simulink model "UAV_3dof_Autonomus"  (R2024b)
settings: Solver=FixedStepDiscrete  StartTime=0.0  StopTime=180  FixedStep=0.05  RelTol=1e-3
settings Model: Creator=ninadbhave  LastModifiedBy=ninadbhave

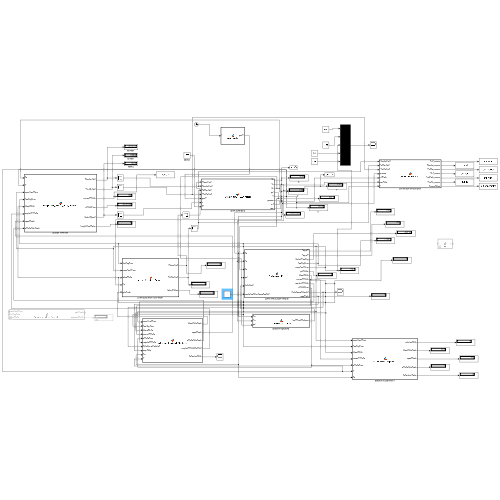
[thumbnail: Simulink's stored preview of the top-level diagram]
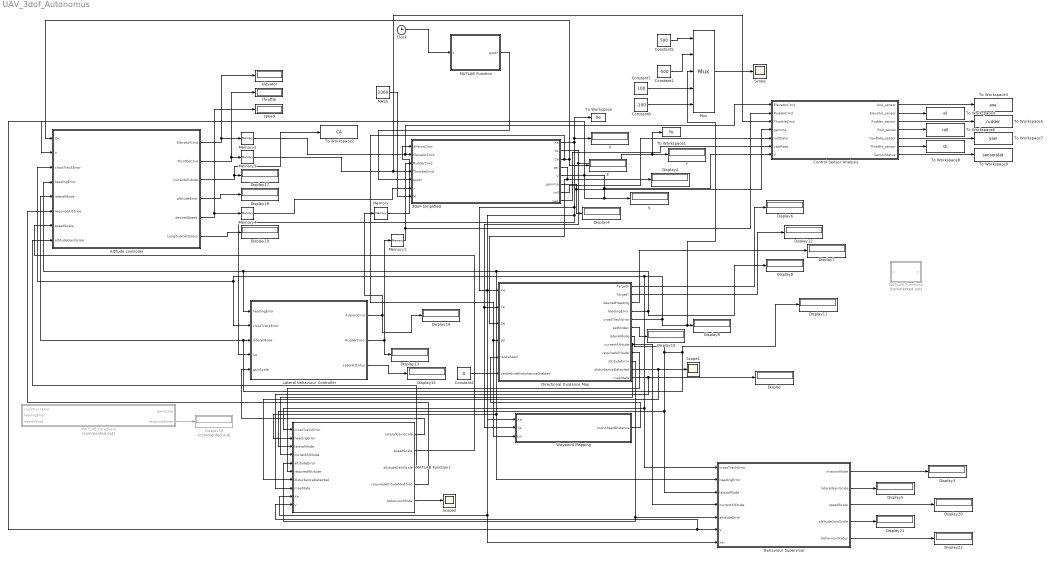
== system UAV_3dof_Autonomus ==
  3DoF-Simplified : MATLAB Function  TreatAsAtomicUnit=on
  Altitude controller : MATLAB Function  TreatAsAtomicUnit=on
  Behaviour Supervisor : MATLAB Function  TreatAsAtomicUnit=on
  Clock : Clock
  Constant1 : Constant  Value=-500
  Constant2 : Constant  Value=0
  Constant5 : Constant  Value=500
  Constant7 : Constant  Value=100
  Constant8 : Constant  Value=-100
  Control Sensor Analysis : MATLAB Function  TreatAsAtomicUnit=on
  Directional Guidance Map : MATLAB Function  TreatAsAtomicUnit=on
  Display{,2..15,17..22} (21 alike) : Display
  Display16 : Display  Commented=on
  Lateral behaviour Controller : MATLAB Function  TreatAsAtomicUnit=on
  MASS : Constant  Value=1000
  MATLAB Function : MATLAB Function  TreatAsAtomicUnit=on
  MATLAB Function1 : MATLAB Function  TreatAsAtomicUnit=on
  MATLAB Function2 : MATLAB Function  Commented=on  TreatAsAtomicUnit=on
  MATLAB Function4 : MATLAB Function  Commented=on  TreatAsAtomicUnit=on
  Memory : Memory
  Memory1 : Memory
  Memory2 : Memory  InitialCondition=-0.003
  Memory3 : Memory  InitialCondition=0.55
  Memory4 : Memory  InitialCondition=45
  Mux : Mux  Inputs=5
  Scope : Scope
  Scope1 : Scope
  Scope2 : Scope
  To Workspace : ToWorkspace  VariableName=Xe  SaveFormat=Timeseries  SampleTime=-1
  To Workspace1 : ToWorkspace  VariableName=Ye  SaveFormat=Timeseries  SampleTime=-1
  To Workspace2 : ToWorkspace  VariableName=CA  SaveFormat=Timeseries  SampleTime=-1
  To Workspace3 : ToWorkspace  VariableName=aoa  SaveFormat=Timeseries  SampleTime=-1
  To Workspace4 : ToWorkspace  VariableName=el  SaveFormat=Timeseries  SampleTime=-1
  To Workspace5 : ToWorkspace  VariableName=rudder  SaveFormat=Timeseries  SampleTime=-1
  To Workspace6 : ToWorkspace  VariableName=roll  SaveFormat=Timeseries  SampleTime=-1
  To Workspace7 : ToWorkspace  VariableName=yaw  SaveFormat=Timeseries  SampleTime=-1
  To Workspace8 : ToWorkspace  VariableName=th  SaveFormat=Timeseries  SampleTime=-1
  To Workspace9 : ToWorkspace  VariableName=sensorstat  SaveFormat=Timeseries  SampleTime=-1
  V : Display
  Waypoint Mapping : MATLAB Function  TreatAsAtomicUnit=on
  X : Display
  Y : Display
  Z : Display
  elevator : Display
  speed : Display
  throttle : Display
  wires:
  MATLAB Function/1(gustY) -> 3DoF-Simplified/5(gustY)
  3DoF-Simplified/1(Xe) -> MATLAB Function1/9(Xe), Behaviour Supervisor/7(Xe), Lateral behaviour Controller/4(Xe), Waypoint Mapping/1(Xe), Directional Guidance Map/1(Xe), To Workspace/1, X/1
  3DoF-Simplified/6(gamma) -> Display4/1, Control Sensor Analysis/4(gamma)
  3DoF-Simplified/5(V) -> MATLAB Function1/10(V), Behaviour Supervisor/6(V), Control Sensor Analysis/7(V), V/1, Altitude controller/2(V)
  3DoF-Simplified/4(psi) -> Display2/1, Waypoint Mapping/3(psi), Directional Guidance Map/4(psi)
  3DoF-Simplified/3(Ze) -> Directional Guidance Map/3(Ze), Z/1, Altitude controller/1(Ze)
  3DoF-Simplified/2(Ye) -> To Workspace1/1, Y/1, Waypoint Mapping/2(Ye), Directional Guidance Map/2(Ye)
  Directional Guidance Map/1(TargetX) -> Display6/1
  Directional Guidance Map/7(lateralMode) -> Behaviour Supervisor/3(lateralMode), MATLAB Function1/3(lateralMode), Display11/1, Altitude controller/5(lateralMode), Lateral behaviour Controller/3(lateralMode)
  Directional Guidance Map/6(pathIndex) -> Display10/1
  Directional Guidance Map/5(crossTrackError) -> Lateral behaviour Controller/2(crossTrackError), Altitude controller/3(crossTrackError), Behaviour Supervisor/1(crossTrackError), MATLAB Function1/1(crossTrackError), Mux/3, Display9/1
  Directional Guidance Map/4(headingError) -> Altitude controller/4(headingError), Lateral behaviour Controller/1(headingError), Behaviour Supervisor/2(headingError), MATLAB Function1/2(headingError), Display8/1
  Directional Guidance Map/3(desiredHeading) -> Display7/1
  Directional Guidance Map/2(TargetY) -> Display12/1
  Lateral behaviour Controller/1(AileronCmd) -> Display14/1, Memory/1
  Lateral behaviour Controller/2(RudderCmd) -> Display13/1, Memory1/1
  Memory/1 -> 3DoF-Simplified/1(AileronCmd)
  Memory1/1 -> 3DoF-Simplified/3(RudderCmd), Control Sensor Analysis/2(RudderCmd)
  Lateral behaviour Controller/3(LateralStatus) -> Display15/1
  Waypoint Mapping/1(lookAheadDistance) -> Directional Guidance Map/5(lookahead)
  Constant5/1 -> Mux/1
  Mux/1 -> Scope/1
  Constant1/1 -> Mux/2
  MATLAB Function4/2(responseMode) -> Display16/1
  Constant7/1 -> Mux/4
  Constant8/1 -> Mux/5
  Altitude controller/3(currentAltitude) -> To Workspace2/1, Display17/1
  Altitude controller/4(altitudeError) -> Display18/1
  Altitude controller/6(LongitudinalStatus) -> Display19/1
  Altitude controller/1(ElevatorCmd) -> elevator/1, Memory2/1
  Memory2/1 -> Control Sensor Analysis/1(ElevatorCmd), 3DoF-Simplified/2(ElevatorCmd)
  Altitude controller/2(ThrottleCmd) -> throttle/1, Memory3/1
  Memory3/1 -> 3DoF-Simplified/4(ThrottleCmd), Control Sensor Analysis/3(ThrottleCmd)
  Altitude controller/5(desiredSpeed) -> speed/1, Memory4/1
  Memory4/1 -> 3DoF-Simplified/6(v)
  MASS/1 -> 3DoF-Simplified/7(M)
  Clock/1 -> MATLAB Function/1(t)
  3DoF-Simplified/7(roll) -> Control Sensor Analysis/5(rollState)
  3DoF-Simplified/8(yaw) -> Control Sensor Analysis/6(yawRate)
  Control Sensor Analysis/1(AoA_sensor) -> To Workspace3/1
  Control Sensor Analysis/2(Elevator_sensor) -> To Workspace4/1
  Control Sensor Analysis/3(Rudder_sensor) -> To Workspace5/1
  Control Sensor Analysis/4(Roll_sensor) -> To Workspace6/1
  Control Sensor Analysis/5(YawRate_sensor) -> To Workspace7/1
  Control Sensor Analysis/6(Throttle_sensor) -> To Workspace8/1
  Control Sensor Analysis/7(SensorStatus) -> To Workspace9/1
  Constant2/1 -> Directional Guidance Map/6(centrelineDisturbanceEnabled)
  Directional Guidance Map/12(mapState) -> MATLAB Function1/8(mapState), Display/1
  Directional Guidance Map/8(currentAltitude) -> MATLAB Function1/4(currentAltitude), Behaviour Supervisor/4(currentAltitude)
  Directional Guidance Map/10(altitudeError) -> MATLAB Function1/5(altitudeError), Behaviour Supervisor/5(altitudeError)
  Directional Guidance Map/9(requiredAltitude) -> MATLAB Function1/6(requiredAltitude)
  Directional Guidance Map/11(disturbanceDetected) -> MATLAB Function1/7(disturbanceDetected), Scope1/1
  Behaviour Supervisor/1(missionMode) -> Display3/1
  Behaviour Supervisor/2(lateralGainScale) -> Display5/1
  Behaviour Supervisor/3(speedScale) -> Display20/1
  Behaviour Supervisor/4(altitudeGainScale) -> Display21/1
  Behaviour Supervisor/5(behaviourStatus) -> Display22/1
  MATLAB Function1/1(lateralGainScale) -> Lateral behaviour Controller/5(gainScale)
  MATLAB Function1/4(requiredAltitudeModified) -> Altitude controller/6(requiredAltitude)
  MATLAB Function1/3(altitudeGainScale) -> Altitude controller/8(altitudeGainScale)
  MATLAB Function1/2(speedScale) -> Altitude controller/7(speedScale)
  MATLAB Function1/5(behaviourMode) -> Scope2/1

== matlab function UAV_3dof_Autonomus/MATLAB Function ==
  data: t input; gustY output
function gustY = Gust_Model(t)
%#codegen
% Gust_Model
%
% Time-based lateral gust disturbance model.
%
% Unit:
%   gustY is lateral gust velocity in m/s.
%
% Conversion:
%   10 km/h = 2.78 m/s
%   15 km/h = 4.17 m/s

gustY = 0;

% 10 km/h lateral gust
if t >= 30 && t < 45
    gustY = 2.78;

% 10 km/h lateral gust in opposite direction
elseif t >= 65 && t < 80
    gustY = -2.78;

% 15 km/h short stronger gust
elseif t >= 95 && t < 100
    gustY = 4.17;
end

end

== matlab function UAV_3dof_Autonomus/Control Sensor Analysis ==
  data: ElevatorCmd input; AoA_sensor output; RudderCmd input; ThrottleCmd input; gamma input; rollState input; yawRate input; V input; Elevator_sensor output; Rudder_sensor output; Roll_sensor output; YawRate_sensor output; Throttle_sensor output; SensorStatus output
function [AoA_sensor, Elevator_sensor, Rudder_sensor, Roll_sensor, YawRate_sensor, Throttle_sensor, SensorStatus] = Virtual_Sensor_Pack(ElevatorCmd, RudderCmd, ThrottleCmd, gamma, rollState, yawRate, V)
%#codegen
% Virtual_Sensor_Pack
%
% Creates virtual telemetry sensor outputs for post-simulation analysis.
%
% These are not high-fidelity physical sensors.
% They are simplified monitoring channels derived from plant/controller states.

%% Sensor outputs

Elevator_sensor = ElevatorCmd;
Rudder_sensor = RudderCmd;
Throttle_sensor = ThrottleCmd;

Roll_sensor = rollState;
YawRate_sensor = yawRate;

%% Simplified AoA estimate
% In a full aircraft model:
%   AoA = pitch angle - flight path angle
%
% This simplified 3DOF model does not explicitly track pitch angle.
% Therefore, AoA is estimated from elevator command and flight path angle.
%
% Negative elevator usually increases climb tendency / effective AoA.

K_elev_to_aoa = 4.0;   % rad per elevator command unit, simplified estimate

AoA_sensor = -K_elev_to_aoa * ElevatorCmd - gamma;

%% Safety / sensor status logic

SensorStatus = 1;   % normal

% AoA caution threshold
if abs(AoA_sensor) > 0.25
    SensorStatus = 2;   % AoA caution
end

% Excessive roll condition
if abs(Roll_sensor) > 0.8
    SensorStatus = 3;   % roll caution
end

% Excessive yaw-rate condition
if abs(YawRate_sensor) > 0.6
    SensorStatus = 4;   % yaw-rate caution
end

% Low speed condition
if V < 45
    SensorStatus = 5;   % low-speed caution
end

end

== matlab function UAV_3dof_Autonomus/Behaviour Supervisor ==
  data: crossTrackError input; missionMode output; headingError input; lateralMode input; currentAltitude input; altitudeError input; V input; Xe input; lateralGainScale output; speedScale output; altitudeGainScale output; behaviourStatus output
function [missionMode, lateralGainScale, speedScale, altitudeGainScale, behaviourStatus] = AI_Behaviour_Supervisor(crossTrackError, headingError, lateralMode, currentAltitude, altitudeError, V, Xe)
%#codegen
% AI_Behaviour_Supervisor
%
% Closed-loop behavioural supervisor for the autonomous UAV model.
%
% This block observes path tracking, altitude hold and speed condition,
% then adjusts controller scaling factors.
%
% missionMode:
%   1 = normal valley following
%   2 = lateral recovery / caution
%   3 = altitude priority
%   4 = mission end / safe exit
%
% Scaling outputs:
%   lateralGainScale   -> modifies lateral correction authority
%   speedScale         -> modifies desired speed
%   altitudeGainScale  -> modifies altitude-hold authority

%% Absolute values

absCTE = abs(crossTrackError);
absHeadingError = abs(headingError);
absAltitudeError = abs(altitudeError);

%% Defaults

missionMode = 1;
lateralGainScale = 1.0;
speedScale = 1.0;
altitudeGainScale = 1.0;
behaviourStatus = 1;

finalWaypointX = 7700;

%% Behaviour decisions

if Xe >= finalWaypointX

    % End of mapped mission route
    missionMode = 4;
    lateralGainScale = 0.85;
    speedScale = 0.90;
    altitudeGainScale = 1.0;
    behaviourStatus = 4;

elseif absCTE > 500

    % Outside safe corridor: strong lateral recovery
    missionMode = 2;
    lateralGainScale = 1.15;
    speedScale = 0.86;
    altitudeGainScale = 0.75;
    behaviourStatus = 2;

elseif absCTE > 250 || lateralMode == 2 || absHeadingError > 0.20

    % Outside preferred corridor or strong correction
    missionMode = 2;
    lateralGainScale = 1.08;
    speedScale = 0.92;
    altitudeGainScale = 0.85;
    behaviourStatus = 2;

elseif absAltitudeError > 15

    % Lateral is acceptable, altitude needs attention
    missionMode = 3;
    lateralGainScale = 0.96;
    speedScale = 0.97;
    altitudeGainScale = 1.08;
    behaviourStatus = 3;

else

    % Normal autonomous valley following
    missionMode = 1;
    lateralGainScale = 1.0;
    speedScale = 1.0;
    altitudeGainScale = 1.0;
    behaviourStatus = 1;

end

%% Low-altitude protection

if currentAltitude < 70
    missionMode = 3;
    lateralGainScale = 0.90;
    speedScale = 0.90;
    altitudeGainScale = 1.15;
    behaviourStatus = 3;
end

%% Overspeed protection

if V > 75
    speedScale = speedScale * 0.95;
end

%% Final bounds

if lateralGainScale > 1.20
    lateralGainScale = 1.20;
elseif lateralGainScale < 0.80
    lateralGainScale = 0.80;
end

if speedScale > 1.00
    speedScale = 1.00;
elseif speedScale < 0.80
    speedScale = 0.80;
end

if altitudeGainScale > 1.20
    altitudeGainScale = 1.20;
elseif altitudeGainScale < 0.70
    altitudeGainScale = 0.70;
end

end

== matlab function UAV_3dof_Autonomus/MATLAB Function2 ==
  data: u input; y output
function y = fcn(u)

y = u;

== matlab function UAV_3dof_Autonomus/MATLAB Function1 ==
  data: crossTrackError input; lateralGainScale output; headingError input; lateralMode input; currentAltitude input; altitudeError input; requiredAltitude input; disturbanceDetected input; mapState input; Xe input; V input; speedScale output; altitudeGainScale output; requiredAltitudeModified output; behaviourMode output
function [lateralGainScale, speedScale, altitudeGainScale, requiredAltitudeModified, behaviourMode] = Behaviour_Feedback_Controller(crossTrackError, headingError, lateralMode, currentAltitude, altitudeError, requiredAltitude, disturbanceDetected, mapState, Xe, V)
%#codegen
% Behaviour_Feedback_Controller
%
% Supervisory feedback controller for autonomous UAV behaviour.
%
% It receives map-state information, UAV tracking errors and aircraft state.
% It then modifies controller gains and the altitude reference.
%
% behaviourMode:
%   1 = normal valley following
%   2 = disturbed centreline / escape-climb behaviour
%   3 = lateral recovery
%   4 = mission complete

%% Defaults

lateralGainScale = 1.0;
speedScale = 1.0;
altitudeGainScale = 1.0;
requiredAltitudeModified = requiredAltitude;
behaviourMode = 1;

%% Absolute error values

absCTE = abs(crossTrackError);
absHeadingError = abs(headingError);
absAltitudeError = abs(altitudeError);

finalWaypointX = 7700;

%% Behaviour decision logic

if Xe >= finalWaypointX

    % End of mapped route
    behaviourMode = 4;

    lateralGainScale = 0.85;
    speedScale = 0.90;
    altitudeGainScale = 1.00;
    requiredAltitudeModified = requiredAltitude;

elseif disturbanceDetected >= 0.5 || mapState == 2

    % Centreline disturbed: reject normal path and prioritise climb
    behaviourMode = 2;

    requiredAltitudeModified = 1000;

    lateralGainScale = 1.05;
    speedScale = 0.88;
    altitudeGainScale = 1.20;

elseif absCTE > 250 || lateralMode == 2 || absHeadingError > 0.20

    % Lateral recovery mode
    behaviourMode = 3;

    requiredAltitudeModified = requiredAltitude;

    lateralGainScale = 1.12;
    speedScale = 0.92;
    altitudeGainScale = 0.90;

else

    % Normal valley following
    behaviourMode = 1;

    requiredAltitudeModified = requiredAltitude;

    lateralGainScale = 1.00;
    speedScale = 1.00;
    altitudeGainScale = 1.00;

end

%% Low-altitude protection

if currentAltitude < 70

    behaviourMode = 2;

    if requiredAltitudeModified < 1000
        requiredAltitudeModified = 1000;
    end

    lateralGainScale = 0.95;
    speedScale = 0.88;
    altitudeGainScale = 1.20;

end

%% Large altitude-error response

if absAltitudeError > 100

    altitudeGainScale = altitudeGainScale + 0.05;
    speedScale = speedScale * 0.96;

end

%% Overspeed protection

if V > 75

    speedScale = speedScale * 0.95;

end

%% Saturation limits

if lateralGainScale > 1.20
    lateralGainScale = 1.20;
elseif lateralGainScale < 0.80
    lateralGainScale = 0.80;
end

if speedScale > 1.00
    speedScale = 1.00;
elseif speedScale < 0.80
    speedScale = 0.80;
end

if altitudeGainScale > 1.25
    altitudeGainScale = 1.25;
elseif altitudeGainScale < 0.70
    altitudeGainScale = 0.70;
end

end

== matlab function UAV_3dof_Autonomus/Directional Guidance Map ==
  data: Xe input; TargetX output; Ye input; Ze input; psi input; TargetY output; desiredHeading output; headingError output; crossTrackError output; pathIndex output; lateralMode output; lookahead input; centrelineDisturbanceEnabled input; currentAltitude output; requiredAltitude output; altitudeError output; disturbanceDetected output; mapState output
function [TargetX, TargetY, desiredHeading, headingError, crossTrackError, pathIndex, lateralMode, currentAltitude, requiredAltitude, altitudeError, disturbanceDetected, mapState] = Environment_Map(Xe, Ye, Ze, psi, lookahead, centrelineDisturbanceEnabled)
%#codegen
% Environment_Map
%
% Two-state behavioural environment map with external disturbance enable input.
%
% Inputs:
%   Xe, Ye, Ze, psi, lookahead
%   centrelineDisturbanceEnabled:
%       0 = centreline clear / normal valley following
%       1 = disturbance enabled / reject centreline in disturbance zone
%
% mapState:
%   1 = centreline clear / normal valley-following
%   2 = centreline disturbed / straight escape path

%% 1. Valley centreline waypoints

waypoints = [ ...
     300   -300;
    1600    300;
    3000   -450;
    4500    200;
    6000   -300;
    7700    350];

wpX = waypoints(:,1);
wpY = waypoints(:,2);

numWP = size(waypoints,1);

%% 2. Behaviour parameters

disturbanceStartX = 3300;
disturbanceEndX   = 4700;

normalMissionAltitude = 100;
safeEscapeAltitude    = 1000;

escapeOffsetY = 500;
escapeSide = 1;

%% 3. Clamp Xe inside map range

Xe_clamped = Xe;

if Xe_clamped < wpX(1)
    Xe_clamped = wpX(1);
elseif Xe_clamped > wpX(end)
    Xe_clamped = wpX(end);
end

%% 4. Active path segment

pathIndex = 1;

for i = 1:(numWP-1)
    if Xe_clamped >= wpX(i) && Xe_clamped < wpX(i+1)
        pathIndex = i;
    end
end

if Xe_clamped >= wpX(end)
    pathIndex = numWP - 1;
end

%% 5. Normal curved valley reference

normalPathY = interp1(wpX, wpY, Xe_clamped, 'pchip');

%% 6. Two-state behavioural map selection

mapState = 1;
disturbanceDetected = 0;
requiredAltitude = normalMissionAltitude;

pathY = normalPathY;

currentAltitude = -Ze;

disturbanceMidX = 0.5 * (disturbanceStartX + disturbanceEndX);
disturbanceMidY = interp1(wpX, wpY, disturbanceMidX, 'pchip');

escapeLineY = disturbanceMidY + escapeSide * escapeOffsetY;

% Altitude at which the UAV is allowed to commit to lateral escape.
% For a full real vehicle this could be close to 1000 m.
% For this simulation, use a lower threshold so the behaviour is visible.
escapeCommitAltitude = 170;

if centrelineDisturbanceEnabled >= 0.5

    if Xe_clamped >= disturbanceStartX && Xe_clamped <= disturbanceEndX

        disturbanceDetected = 1;
        requiredAltitude = safeEscapeAltitude;

        if centrelineDisturbanceEnabled >= 1.5

            % Severe disturbance mode:
            % Do not immediately ditch the path.
            % First prioritise climb. Only escape laterally once altitude is safer.

            if currentAltitude < escapeCommitAltitude

                mapState = 2;          % climb-priority disturbance mode
                pathY = normalPathY;   % keep path stable while climbing

            else

                mapState = 3;          % lateral escape permitted
                pathY = escapeLineY;   % ditch centreline only after gaining altitude

            end

        else

            % Standard disturbance mode:
            % Direct escape behaviour.
            mapState = 3;
            pathY = escapeLineY;

        end

    else

        mapState = 1;
        disturbanceDetected = 0;
        requiredAltitude = normalMissionAltitude;
        pathY = normalPathY;

    end

else

    mapState = 1;
    disturbanceDetected = 0;
    requiredAltitude = normalMissionAltitude;
    pathY = normalPathY;

end

%% 7. Cross-track error based on selected reference

crossTrackError = Ye - pathY;

%% 8. Local path tangent

dx = 60;

xBack = Xe_clamped - dx;
xForward = Xe_clamped + dx;

if xBack < wpX(1)
    xBack = wpX(1);
end

if xForward > wpX(end)
    xForward = wpX(end);
end

if mapState == 1

    yBack = interp1(wpX, wpY, xBack, 'pchip');
    yForward = interp1(wpX, wpY, xForward, 'pchip');

else

    yBack = escapeLineY;
    yForward = escapeLineY;

end

localSlope = (yForward - yBack) / (xForward - xBack + 1e-6);

pathHeading = atan(localSlope);
pathHeading = atan2(sin(pathHeading), cos(pathHeading));

%% 9. Lookahead target

if lookahead > 180
    lookahead = 180;
elseif lookahead < 80
    lookahead = 80;
end

TargetX = Xe_clamped + lookahead;

if TargetX > wpX(end)
    TargetX = wpX(end);
elseif TargetX < wpX(1)
    TargetX = wpX(1);
end

if mapState == 1
    TargetY = interp1(wpX, wpY, TargetX, 'pchip');
else
    TargetY = escapeLineY;
end

previewHeading = atan2(TargetY - Ye, TargetX - Xe);
previewHeading = atan2(sin(previewHeading), cos(previewHeading));

%% 10. Cross-track heading correction

K_cte_heading = 0.0065;

cteHeadingCorrection = atan(K_cte_heading * crossTrackError);

if cteHeadingCorrection > 0.65
    cteHeadingCorrection = 0.65;
elseif cteHeadingCorrection < -0.65
    cteHeadingCorrection = -0.65;
end

%% 11. Desired heading

blendPreview = 0.35;

desiredHeading = ...
    (1 - blendPreview) * (pathHeading - cteHeadingCorrection) + ...
    blendPreview * previewHeading;

desiredHeading = atan2(sin(desiredHeading), cos(desiredHeading));

headingError = desiredHeading - psi;
headingError = atan2(sin(headingError), cos(headingError));

%% 12. Lateral mode

absCTE = abs(crossTrackError);
absHeadingError = abs(headingError);

if Xe >= wpX(end)
    lateralMode = 0;

elseif mapState == 2
    lateralMode = 2;

elseif absCTE <= 40 && absHeadingError <= 0.05
    lateralMode = 0;

elseif absCTE <= 120 && absHeadingError <= 0.15
    lateralMode = 1;

else
    lateralMode = 2;
end

%% 13. Altitude outputs

currentAltitude = -Ze;
altitudeError = requiredAltitude - currentAltitude;

end

== matlab function UAV_3dof_Autonomus/3DoF-Simplified ==
  data: AileronCmd input; Xe output; ElevatorCmd input; RudderCmd input; ThrottleCmd input; gustY input; Ye output; Ze output; psi output; V output; gamma output; v input; M input; roll output; yaw output
function [Xe, Ye, Ze, psi, V, gamma, roll, yaw] = Custom_3DOF_UAV_Model(AileronCmd, ElevatorCmd, RudderCmd, ThrottleCmd, gustY, v, M)
% Custom simplified 3DOF UAV model for AI-supervised path following.
%
% Model purpose:
%   Stable conceptual UAV plant for autonomous valley/corridor navigation.
%
% Inputs:
%   AileronCmd   - lateral/roll control command
%   ElevatorCmd  - vertical/climb control command
%   RudderCmd    - yaw/directional control command
%   ThrottleCmd  - throttle command, 0 to 1
%   gustY        - lateral gust disturbance, m/s
%
% Outputs:
%   Xe     - East position, m
%   Ye     - North position, m
%   Ze     - NED vertical position, m. Negative Ze = altitude above ground
%   psi    - heading angle, rad
%   V      - forward speed, m/s
%   gamma  - flight path angle, rad

%% Persistent aircraft states

persistent x y z heading speed flightPathAngle rollState yawRate

dt = 0.05;     % simulation integration step, s

%% Initial conditions

if isempty(x)
    x = 300;                 % initial East position, m
    y = -300;                % initial North position, m
    z = -100;                % NED: altitude = -Ze = 300 m
    heading = 0;             % rad, initially flying along +X
    speed =v;              % initial speed, m/s
    flightPathAngle = 0;     % rad
    rollState = 0;           % simplified bank/roll state, rad
    yawRate = 0;             % rad/s
end

%% Aircraft parameters: 1000 kg reconnaissance UAV style

m = M;       % kg
g = 9.81;       % m/s^2
rho = 1.225;    % kg/m^3

S = 14.0;       % m^2, wing reference area
W = m*g;        % N, weight

% Drag model for forward force balance
CD0 = 0.040;
kD  = 0.055;

% Representative lift coefficient used only for drag estimate
CL_trim = 0.30;

% Propulsion
Tmax = 2600;    % N, conceptual max thrust

%% Input limits

if AileronCmd > 0.08
    AileronCmd = 0.08;
elseif AileronCmd < -0.08
    AileronCmd = -0.08;
end

if ElevatorCmd > 0.08
    ElevatorCmd = 0.08;
elseif ElevatorCmd < -0.25
    ElevatorCmd = -0.25;
end

if RudderCmd > 0.08
    RudderCmd = 0.08;
elseif RudderCmd < -0.08
    RudderCmd = -0.08;
end

if ThrottleCmd > 1
    ThrottleCmd = 1;
elseif ThrottleCmd < 0
    ThrottleCmd = 0;
end

if gustY > 20
    gustY = 20;
elseif gustY < -20
    gustY = -20;
end

%% Forward force balance: Fx = T - D

qbar = 0.5*rho*speed^2;

CD = CD0 + kD*CL_trim^2;
D = qbar*S*CD;

T = Tmax*ThrottleCmd;

Fx = T - D;

speedDot = Fx/m;

speed = speed + speedDot*dt;

if speed < 20
    speed = 20;
elseif speed > 65
    speed = 65;
end

%% Stable vertical dynamics
% This replaces unstable direct lift-based altitude propagation.
% Negative elevator = climb command.
% Positive elevator = descent command.

gammaCommand = -1.2 * ElevatorCmd;

% Limit commanded flight-path angle
if gammaCommand > 0.08
    gammaCommand = 0.08;
elseif gammaCommand < -0.08
    gammaCommand = -0.08;
end

% First-order response toward commanded gamma
gammaDot = 0.8 * (gammaCommand - flightPathAngle);

flightPathAngle = flightPathAngle + gammaDot*dt;

% Limit actual flight-path angle
if flightPathAngle > 0.10
    flightPathAngle = 0.10;
elseif flightPathAngle < -0.10
    flightPathAngle = -0.10;
end

%% Lateral / directional dynamics
% Aileron produces bank/roll response.
% Rudder produces yaw response.
% Gust produces lateral drift and yaw disturbance.

rollDot = 3.2*AileronCmd - 1.8*rollState;

rollState = rollState + rollDot*dt;

if rollState > 0.55
    rollState = 0.55;
elseif rollState < -0.55
    rollState = -0.55;
end

% Coordinated turn approximation
turnRateFromRoll = g*tan(rollState)/speed;

% Rudder and gust contribution
rudderYawEffect = 0.9*RudderCmd;
gustYawEffect   = -0.010*gustY;

yawRateCommand = turnRateFromRoll + rudderYawEffect + gustYawEffect;

% Yaw damping / vertical stabilizer effect
yawRateDot = 1.8*(yawRateCommand - yawRate);

yawRate = yawRate + yawRateDot*dt;

if yawRate > 0.35
    yawRate = 0.35;
elseif yawRate < -0.35
    yawRate = -0.35;
end

heading = heading + yawRate*dt;
heading = atan2(sin(heading), cos(heading));

%% Position update

xDot = speed*cos(flightPathAngle)*cos(heading);
yDot = speed*cos(flightPathAngle)*sin(heading) + gustY;

% NED convention:
% positive gamma = climb = Ze becomes more negative
zDot = -speed*sin(flightPathAngle);

x = x + xDot*dt;
y = y + yDot*dt;
z = z + zDot*dt;

%% Hard altitude safety limit
% Prevents the simple plant from becoming numerically unrealistic.

if z > -50
    z = -50;      % minimum altitude = 50 m
elseif z < -1500
    z = -1500;    % maximum altitude = 1500 m
end

%% Outputs

Xe = x;
Ye = y;
Ze = z;
psi = heading;
V = speed;
gamma = flightPathAngle;
roll = rollState;
yaw = yawRate;
end

== matlab function UAV_3dof_Autonomus/Lateral behaviour Controller ==
  data: headingError input; AileronCmd output; crossTrackError input; lateralMode input; RudderCmd output; Xe input; LateralStatus output; gainScale input
function [AileronCmd, RudderCmd, LateralStatus] = Lateral_Behaviour_Controller(headingError, crossTrackError, lateralMode, Xe, gainScale)
%#codegen
% Centreline-hugging lateral controller
%
% Uses heading error, cross-track error, and cross-track rate damping.
% Designed to force the UAV closer to the black centreline.
 
%% Persistent memory
 
persistent prevAileron prevRudder prevCTE prevHeadingError
 
if isempty(prevAileron)
    prevAileron = 0;
    prevRudder = 0;
    prevCTE = 0;
    prevHeadingError = 0;
end
 
dt = 0.05;
 
%% Input limits
 
if headingError > 0.9
    headingError = 0.9;
elseif headingError < -0.9
    headingError = -0.9;
end
 
if crossTrackError > 700
    crossTrackError = 700;
elseif crossTrackError < -700
    crossTrackError = -700;
end
 
if gainScale > 1.2
    gainScale = 1.2;
elseif gainScale < 0.8
    gainScale = 0.8;
end
 
%% Rates for damping
 
cteRate = (crossTrackError - prevCTE)/dt;
headingRate = (headingError - prevHeadingError)/dt;
 
if cteRate > 220
    cteRate = 220;
elseif cteRate < -220
    cteRate = -220;
end
 
if headingRate > 2.0
    headingRate = 2.0;
elseif headingRate < -2.0
    headingRate = -2.0;
end
 
absCTE = abs(crossTrackError);
absHeading = abs(headingError);
 
%% Status
 
finalWaypointX = 7700;
 
if Xe >= finalWaypointX
    LateralStatus = 5;
 
elseif absCTE > 220
    LateralStatus = 4;      % recovery
 
elseif absCTE > 100 || absHeading > 0.18 || lateralMode == 2
    LateralStatus = 3;      % strong correction
 
elseif absCTE > 40 || absHeading > 0.06 || lateralMode == 1
    LateralStatus = 2;      % mild correction
 
else
    LateralStatus = 1;      % centreline tracking
end
 
%% Centreline-hugging gains
 
if LateralStatus == 1
    K_h_ail = 0.075;
    K_cte_ail = 0.000095;
    K_dcte_ail = 0.000115;
    K_dh_ail = 0.018;
 
    K_h_rud = 0.095;
    K_cte_rud = 0.000120;
    K_dcte_rud = 0.000140;
    K_dh_rud = 0.020;
 
    aileronLimit = 0.045;
    rudderLimit = 0.055;
 
elseif LateralStatus == 2
    K_h_ail = 0.090;
    K_cte_ail = 0.000135;
    K_dcte_ail = 0.000155;
    K_dh_ail = 0.020;
 
    K_h_rud = 0.115;
    K_cte_rud = 0.000165;
    K_dcte_rud = 0.000180;
    K_dh_rud = 0.024;
 
    aileronLimit = 0.060;
    rudderLimit = 0.070;
 
elseif LateralStatus == 3
    K_h_ail = 0.110;
    K_cte_ail = 0.000180;
    K_dcte_ail = 0.000200;
    K_dh_ail = 0.024;
 
    K_h_rud = 0.135;
    K_cte_rud = 0.000220;
    K_dcte_rud = 0.000240;
    K_dh_rud = 0.028;
 
    aileronLimit = 0.075;
    rudderLimit = 0.080;
 
elseif LateralStatus == 4
    K_h_ail = 0.125;
    K_cte_ail = 0.000230;
    K_dcte_ail = 0.000260;
    K_dh_ail = 0.028;
 
    K_h_rud = 0.150;
    K_cte_rud = 0.000270;
    K_dcte_rud = 0.000300;
    K_dh_rud = 0.032;
 
    aileronLimit = 0.080;
    rudderLimit = 0.080;
 
else
    K_h_ail = 0;
    K_cte_ail = 0;
    K_dcte_ail = 0;
    K_dh_ail = 0;
 
    K_h_rud = 0;
    K_cte_rud = 0;
    K_dcte_rud = 0;
    K_dh_rud = 0;
 
    aileronLimit = 0;
    rudderLimit = 0;
end
 
%% Apply only small gain scale
 
K_h_ail = K_h_ail * gainScale;
K_cte_ail = K_cte_ail * gainScale;
 
K_h_rud = K_h_rud * gainScale;
K_cte_rud = K_cte_rud * gainScale;
 
%% Command law
 
cteCorrection = -crossTrackError;
cteRateCorrection = -cteRate;
 
rawAileron = ...
    K_h_ail*headingError + ...
    K_cte_ail*cteCorrection + ...
    K_dcte_ail*cteRateCorrection - ...
    K_dh_ail*headingRate;
 
rawRudder = ...
    K_h_rud*headingError + ...
    K_cte_rud*cteCorrection + ...
    K_dcte_rud*cteRateCorrection - ...
    K_dh_rud*headingRate;
 
%% Raw command saturation
 
if rawAileron > aileronLimit
    rawAileron = aileronLimit;
elseif rawAileron < -aileronLimit
    rawAileron = -aileronLimit;
end
 
if rawRudder > rudderLimit
    rawRudder = rudderLimit;
elseif rawRudder < -rudderLimit
    rawRudder = -rudderLimit;
end
 
%% Smooth commands but allow tighter tracking
 
maxAileronStep = 0.007;
maxRudderStep = 0.007;
 
aileronStep = rawAileron - prevAileron;
rudderStep = rawRudder - prevRudder;
 
if aileronStep > maxAileronStep
    aileronStep = maxAileronStep;
elseif aileronStep < -maxAileronStep
    aileronStep = -maxAileronStep;
end
 
if rudderStep > maxRudderStep
    rudderStep = maxRudderStep;
elseif rudderStep < -maxRudderStep
    rudderStep = -maxRudderStep;
end
 
AileronCmd = prevAileron + aileronStep;
RudderCmd = prevRudder + rudderStep;
 
%% Final plant-compatible limits
 
if AileronCmd > 0.080
    AileronCmd = 0.080;
elseif AileronCmd < -0.080
    AileronCmd = -0.080;
end
 
if RudderCmd > 0.080
    RudderCmd = 0.080;
elseif RudderCmd < -0.080
    RudderCmd = -0.080;
end
 
%% Store previous values
 
prevAileron = AileronCmd;
prevRudder = RudderCmd;
prevCTE = crossTrackError;
prevHeadingError = headingError;
 
end

== matlab function UAV_3dof_Autonomus/Waypoint Mapping ==
  data: Xe input; lookAheadDistance output; Ye input; psi input
function lookAheadDistance = LookAhead_Controller(Xe, Ye, psi)
%#codegen
% LookAhead_Controller
%
% Adaptive look-ahead controller for curved valley path tracking.
%
% Logic:
%   Close to centreline + straight section  -> longer look-ahead
%   Far from centreline or near a bend      -> shorter look-ahead
%
% This acts as the AI-style target prediction layer.
 
%% Valley route waypoints
 
waypoints = [ ...
     300   -300;
    1600    300;
    3000   -450;
    4500    200;
    6000   -300;
    7700    350];
 
wpX = waypoints(:,1);
wpY = waypoints(:,2);
 
numWP = size(waypoints,1);
 
%% Clamp Xe inside route range
 
Xe_clamped = Xe;
 
if Xe_clamped < wpX(1)
    Xe_clamped = wpX(1);
elseif Xe_clamped > wpX(end)
    Xe_clamped = wpX(end);
end
 
%% Find current path segment
 
pathIndex = 1;
 
for i = 1:(numWP-1)
    if Xe_clamped >= wpX(i) && Xe_clamped < wpX(i+1)
        pathIndex = i;
    end
end
 
if Xe_clamped >= wpX(end)
    pathIndex = numWP - 1;
end
 
%% Current centreline position
 
pathY = interp1(wpX, wpY, Xe_clamped, 'pchip');
 
crossTrackError = Ye - pathY;
absCTE = abs(crossTrackError);
 
%% Estimate local path slope
 
dxSlope = 40;   % m
 
xBack = Xe_clamped - dxSlope;
xForward = Xe_clamped + dxSlope;
 
if xBack < wpX(1)
    xBack = wpX(1);
end
 
if xForward > wpX(end)
    xForward = wpX(end);
end
 
yBack = interp1(wpX, wpY, xBack, 'pchip');
yForward = interp1(wpX, wpY, xForward, 'pchip');
 
localSlope = (yForward - yBack)/(xForward - xBack + 1e-6);
absSlope = abs(localSlope);
 
%% Distance to next waypoint / bend
 
nextWaypointX = wpX(pathIndex + 1);
distanceToNextWP = nextWaypointX - Xe_clamped;
 
if distanceToNextWP < 0
    distanceToNextWP = 0;
end
 
%% Base look-ahead from cross-track error
% Requirement target:
%   valley half-width = 500 m
%   desired cross-track control target = ±50 m
 
if absCTE <= 50
    % Very close to centreline: look ahead for smoothness
    lookAheadDistance = 420;
 
elseif absCTE <= 120
    % Slightly outside ideal band: tighten response
    lookAheadDistance = 320;
 
elseif absCTE <= 250
    % Large deviation: look closer to recover
    lookAheadDistance = 230;
 
else
    % Recovery region
    lookAheadDistance = 170;
end
 
%% Bend-based adjustment
% In sharper bends, reduce look-ahead to avoid corner-cutting.
 
if absSlope > 0.45
    lookAheadDistance = lookAheadDistance * 0.65;
elseif absSlope > 0.25
    lookAheadDistance = lookAheadDistance * 0.80;
end
 
%% Waypoint proximity adjustment
% Near waypoint transitions, reduce look-ahead so it does not cut the bend.
 
if distanceToNextWP < 500
    if lookAheadDistance > 240
        lookAheadDistance = 240;
    end
end
 
if distanceToNextWP < 250
    if lookAheadDistance > 180
        lookAheadDistance = 180;
    end
end
 
%% Final limits
 
if lookAheadDistance > 450
    lookAheadDistance = 450;
elseif lookAheadDistance < 140
    lookAheadDistance = 140;
end
 
end

== matlab function UAV_3dof_Autonomus/MATLAB Function4 ==
  data: crossTrackError input; gainScale output; headingError input; lateralMode input; responseMode output
function [gainScale, responseMode] = External_AI_Gain_Controller(crossTrackError, headingError, lateralMode)

%#codegen

% External_AI_Gain_Controller

%

% Gentle supervisory gain controller.

% This block adapts lateral control authority without causing over-correction.
 
absCTE = abs(crossTrackError);

absHeading = abs(headingError);
 
if absCTE <= 50 && absHeading <= 0.05
 
    responseMode = 1;      % close to centreline

    gainScale = 0.85;
 
elseif absCTE <= 120 && absHeading <= 0.12
 
    responseMode = 2;      % mild correction

    gainScale = 0.95;
 
elseif absCTE <= 250 && absHeading <= 0.22
 
    responseMode = 3;      % moderate correction

    gainScale = 1.05;
 
elseif absCTE <= 400
 
    responseMode = 4;      % strong correction

    gainScale = 1.15;
 
else
 
    responseMode = 5;      % recovery

    gainScale = 1.25;
 
end
 
% Very small map-based increase only

if lateralMode == 2

    gainScale = gainScale * 1.02;

end
 
% Hard safety cap

if gainScale > 1.25

    gainScale = 1.25;

elseif gainScale < 0.80

    gainScale = 0.80;

end
 
end

== matlab function UAV_3dof_Autonomus/Altitude controller ==
  data: Ze input; V input; crossTrackError input; headingError input; lateralMode input; requiredAltitude input; ElevatorCmd output; ThrottleCmd output; currentAltitude output; altitudeError output; desiredSpeed output; LongitudinalStatus output; speedScale input; altitudeGainScale input
function [ElevatorCmd, ThrottleCmd, currentAltitude, altitudeError, desiredSpeed, LongitudinalStatus] = Longitudinal_Altitude_Hold_Controller(Ze, V, crossTrackError, headingError, lateralMode, requiredAltitude, speedScale, altitudeGainScale)
%#codegen
% Longitudinal_Altitude_Hold_Controller
%
% Supervisory-compatible longitudinal controller.
%
% Inputs:
%   Ze                  - NED vertical position from UAV plant
%   V                   - UAV speed
%   crossTrackError     - lateral tracking error
%   headingError        - heading tracking error
%   lateralMode         - lateral guidance mode
%   requiredAltitude    - altitude command from Behaviour Feedback Controller
%   speedScale          - behaviour-loop speed scaling factor
%   altitudeGainScale   - behaviour-loop altitude gain scaling factor
%
% Outputs:
%   ElevatorCmd         - elevator command
%   ThrottleCmd         - throttle command
%   currentAltitude     - current altitude above ground/reference
%   altitudeError       - altitude command error
%   desiredSpeed        - commanded speed after behaviour scaling
%   LongitudinalStatus  - status code
%
% Status:
%   1 = altitude hold normal
%   2 = climb required
%   3 = descend/reduce climb required
%   4 = lateral priority active
%   5 = escape-climb/high-altitude command active

%% Persistent memory

persistent prevElevator prevThrottle prevAltError integralSpeedError

if isempty(prevElevator)
    prevElevator = 0.000;
    prevThrottle = 0.70;
    prevAltError = 0;
    integralSpeedError = 0;
end

%% Time step

dt = 0.05;

%% Convert NED altitude

currentAltitude = -Ze;

%% Protect incoming behaviour-loop inputs

if speedScale > 1.00
    speedScale = 1.00;
elseif speedScale < 0.80
    speedScale = 0.80;
end

if altitudeGainScale > 1.25
    altitudeGainScale = 1.25;
elseif altitudeGainScale < 0.70
    altitudeGainScale = 0.70;
end

%% Mission altitude command from behaviour controller

missionAltitude = requiredAltitude;

% Safety bounds on command altitude
if missionAltitude > 1000
    missionAltitude = 1000;
elseif missionAltitude < 80
    missionAltitude = 80;
end

altitudeError = missionAltitude - currentAltitude;

%% Limit altitude error used by controller

if altitudeError > 300
    altitudeError = 300;
elseif altitudeError < -300
    altitudeError = -300;
end

%% Altitude error rate

altErrorRate = (altitudeError - prevAltError) / dt;

if altErrorRate > 50
    altErrorRate = 50;
elseif altErrorRate < -50
    altErrorRate = -50;
end

%% Lateral workload estimation

absCTE = abs(crossTrackError);
absHeadingError = abs(headingError);

lateralWorkload = 0;

if absCTE > 500
    lateralWorkload = lateralWorkload + 0.45;
elseif absCTE > 250
    lateralWorkload = lateralWorkload + 0.35;
elseif absCTE > 120
    lateralWorkload = lateralWorkload + 0.20;
end

if absHeadingError > 0.25
    lateralWorkload = lateralWorkload + 0.30;
elseif absHeadingError > 0.15
    lateralWorkload = lateralWorkload + 0.20;
elseif absHeadingError > 0.08
    lateralWorkload = lateralWorkload + 0.10;
end

if lateralMode == 2
    lateralWorkload = lateralWorkload + 0.20;
elseif lateralMode == 1
    lateralWorkload = lateralWorkload + 0.10;
end

if lateralWorkload > 0.85
    lateralWorkload = 0.85;
end

%% Desired speed with behaviour-loop scaling

baseDesiredSpeed = 70 - 3*lateralWorkload;

desiredSpeed = baseDesiredSpeed * speedScale;

if desiredSpeed > 72
    desiredSpeed = 72;
elseif desiredSpeed < 58
    desiredSpeed = 58;
end

%% Altitude controller

% Important:
% Negative elevator = climb tendency in your custom plant.
% Positive elevator = descend/reduce climb tendency.

ElevatorNeutral = 0.000;

Kp_alt_base = 0.00018;
Kd_alt_base = 0.00005;

Kp_alt = Kp_alt_base * altitudeGainScale;
Kd_alt = Kd_alt_base * altitudeGainScale;

rawElevator = ElevatorNeutral ...
              - Kp_alt * altitudeError ...
              + Kd_alt * altErrorRate;

%% Lateral priority softening
% During high lateral workload, soften altitude control slightly
% so the UAV does not overreact in both axes at once.

softeningFactor = 1 - 0.30*lateralWorkload;

if softeningFactor < 0.60
    softeningFactor = 0.60;
end

ElevatorCmd = softeningFactor * rawElevator;

%% Elevator saturation

if ElevatorCmd > 0.030
    ElevatorCmd = 0.030;
elseif ElevatorCmd < -0.030
    ElevatorCmd = -0.030;
end

%% Elevator rate limit

maxElevatorStep = 0.0030;

elevatorStep = ElevatorCmd - prevElevator;

if elevatorStep > maxElevatorStep
    elevatorStep = maxElevatorStep;
elseif elevatorStep < -maxElevatorStep
    elevatorStep = -maxElevatorStep;
end

ElevatorCmd = prevElevator + elevatorStep;

%% Speed / throttle controller

speedError = desiredSpeed - V;

if speedError > 25
    speedError = 25;
elseif speedError < -25
    speedError = -25;
end

Kp_speed = 0.010;
Ki_speed = 0.0010;

integralSpeedError = integralSpeedError + speedError * dt;

if integralSpeedError > 35
    integralSpeedError = 35;
elseif integralSpeedError < -35
    integralSpeedError = -35;
end

rawThrottle = 0.70 + Kp_speed * speedError + Ki_speed * integralSpeedError;

%% Add small climb-support throttle
% If the behaviour controller commands a high altitude, give throttle support.

if missionAltitude > 300 && altitudeError > 50
    rawThrottle = rawThrottle + 0.05;
end

%% Throttle saturation

if rawThrottle > 0.90
    rawThrottle = 0.90;
elseif rawThrottle < 0.45
    rawThrottle = 0.45;
end

%% Throttle rate limit

maxThrottleStep = 0.005;

throttleStep = rawThrottle - prevThrottle;

if throttleStep > maxThrottleStep
    throttleStep = maxThrottleStep;
elseif throttleStep < -maxThrottleStep
    throttleStep = -maxThrottleStep;
end

ThrottleCmd = prevThrottle + throttleStep;

%% Longitudinal status logic

if missionAltitude >= 900
    LongitudinalStatus = 5;      % escape-climb/high-altitude command

elseif lateralWorkload > 0.55
    LongitudinalStatus = 4;      % lateral priority active

elseif abs(altitudeError) <= 10
    LongitudinalStatus = 1;      % normal altitude hold

elseif altitudeError > 10
    LongitudinalStatus = 2;      % climb required

else
    LongitudinalStatus = 3;      % descend/reduce climb required
end

%% Update persistent states

prevElevator = ElevatorCmd;
prevThrottle = ThrottleCmd;
prevAltError = altitudeError;

end
